simulink model "tracking"  (R2022a)
settings: Solver=FixedStepDiscrete  StartTime=0.0  StopTime=Traj.duration  RelTol=1e-3  EnableMultiTasking=on
InitFcn:
  | run('busObjects.m')
model workspace (MAT data in the model file):
  omega = 8
  zeta = 0.05
libraries: aru_toolbox x1
settings Model: SimulationMode=external  Creator=Mechatronics  LastModifiedBy=Mechatronics
settings SolverCC: ConcurrentTasks=on  AlgebraicLoopSolver=TrustRegion  PositivePriorityOrder=on  InsertRTBMode=Never (minimum delay)
settings DataIOCC: SaveFormat=Array  SaveState=on  SignalLoggingName=logsOut
settings OptimizationCC: BlockReduction=off  BooleanDataType=off  OptimizeBlockIOStorage=off  BufferReuse=off  GlobalBufferReuse=off  ExpressionFolding=off  LocalBlockOutputs=off  InitFltsAndDblsToZero=on  OptimizeDataStoreBuffers=off  BusAssignmentInplaceUpdate=off
settings DebuggingCC: SaveWithParameterizedLinksMsg=none  UnderspecifiedInitializationDetection=Classic  MergeDetectMultiDrivingBlocksExec=none  CheckExecutionContextPreStartOutputMsg=on  SignalResolutionControl=TryResolveAllWithWarning  TasksWithSamePriorityMsg=none  UnconnectedInputMsg=warning  UnconnectedOutputMsg=warning  UnconnectedLineMsg=warning  SFUnexpectedBacktrackingDiag=warning  SFNoUnconditionalDefaultTransitionDiag=warning  SFExecutionAtInitializationDiag=none  SFMachineParentedDataDiag=warning  ArithmeticOperatorsInVariantConditions=warning
settings HardwareCC: ProdBitPerLong=64  ProdLongLongMode=on  ProdHWDeviceType=Intel->x86-64 (Linux 64)
settings ModelReferenceCC: PropagateSignalLabelsOutOfModel=off
settings SFSimCC: SimUseLocalCustomCode=off  SimTargetLang=C++
settings RTWCC: Description=Simulink Real-Time  SystemTargetFile=slrealtime.tlc  TemplateMakefile=slrealtime_default_tmf  RTWUseLocalCustomCode=off  Toolchain=Simulink Real-Time Toolchain  BuildConfiguration=Faster Runs  CodeExecutionProfiling=on  TargetLang=C++  DLArmComputeVersion=19.05
settings CodeAppCC: StateflowObjectComments=on
settings SimulinkRealTimeTargetCC: MATLABClassNameForMDSCustomization=Simulink.SoftwareTarget.GRTCustomization  UseGCCFastMath=on
settings ConfigComp: CovMetricSettings=dw  CovSaveCumulativeToWorkspaceVar=on  CovSaveSingleToWorkspaceVar=on  CovExternalEMLEnable=off  CovSFcnEnable=off

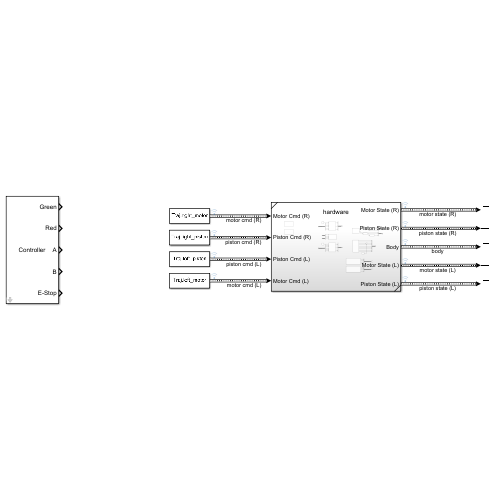
[thumbnail: Simulink's stored preview of the top-level diagram]
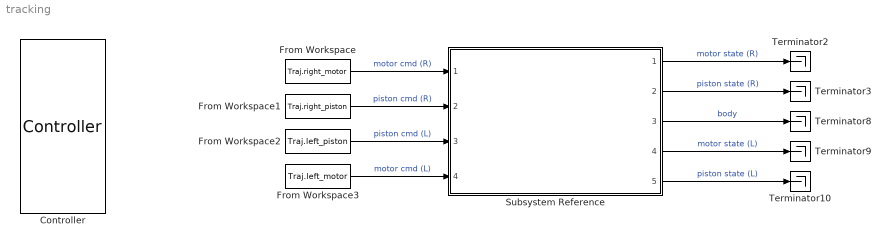
== system tracking ==
  Controller : aru_toolbox/Controller
      link override "LVTTL digital input ": parInternalModuleId=1
      settings: SourceProductName=ARU Toolbox
  From Workspace : FromWorkspace  VariableName=Traj.right_motor  OutDataTypeStr=Bus: MotorCmd  SampleTime=0.001  OutputAfterFinalValue=Holding final value
  From Workspace1 : FromWorkspace  VariableName=Traj.right_piston  OutDataTypeStr=Bus: PistonCmd  SampleTime=0.001  OutputAfterFinalValue=Setting to zero
  From Workspace2 : FromWorkspace  VariableName=Traj.left_piston  OutDataTypeStr=Bus: PistonCmd  SampleTime=0.001  OutputAfterFinalValue=Setting to zero
  From Workspace3 : FromWorkspace  VariableName=Traj.left_motor  OutDataTypeStr=Bus: MotorCmd  SampleTime=0.001  OutputAfterFinalValue=Holding final value
  Subsystem Reference : Subsystem  ReferencedSubsystem=hardware
  Terminator{2..3,8..10} (5 alike) : Terminator
  wires:
  From Workspace/1 -> Subsystem Reference/1  "motor cmd (R)"
  Subsystem Reference/4 -> Terminator9/1  "motor state (L)"
  Subsystem Reference/5 -> Terminator10/1  "piston state (L)"
  Subsystem Reference/3 -> Terminator8/1  "body"
  Subsystem Reference/2 -> Terminator3/1  "piston state (R)"
  Subsystem Reference/1 -> Terminator2/1  "motor state (R)"
  From Workspace3/1 -> Subsystem Reference/4  "motor cmd (L)"
  From Workspace1/1 -> Subsystem Reference/2  "piston cmd (R)"
  From Workspace2/1 -> Subsystem Reference/3  "piston cmd (L)"
